simulink model "AR_Drone_Flight_Control"  (R2014a)
settings: configuration reference "AR_Drone_ConfigSet" (kept outside this file)
values from neighbouring files (symbols this model uses):
  Accelerometer_quick_calibration = [0.003485 0.008674 -0.9985]    [Calibration_Parameters.mat]
  Gyrometer_quick_calibration = [-10.63 2.778 -0.1868]    [Calibration_Parameters.mat]
undefined symbols (not defined in the file or in its folder): Accelerometer_360deg_calibration, Drone_StateModeType, Magnetometer_calibration, Navigation, Navigation_KF_Lib, sigbuilder_block
libraries: simulink x15, vrlib x7, aerolibtransform2 x5, AR_Drone_2_Library x4, dspnetwork x3, aerolibutil x2
(part 3 of 3)

== system AR_Drone_Flight_Control/Navigation/Data Conversion and Measurement Calculation/Calculate Gravity Vector/Calibration_GainOffset ==
  Pre : Inport
  Accel_Calib_Gain : Constant  Value=Accelerometer_360deg_calibration.Gains
      settings: AttributesFormatString=%<Value>
  Accel_Calib_Offset : Constant  Value=Accelerometer_360deg_calibration.Offsets
      settings: AttributesFormatString=%<Value>
  Gain : Gain  Gain=-1  OutDataTypeStr=Inherit: Same as input
  Multiply : Product  Inputs=*/
  Sum : Sum  Inputs=|+-
  Post : Outport
  wires:
  Gain/1 -> Multiply/2
  Accel_Calib_Gain/1 -> Gain/1
  Pre/1 -> Sum/1
  Sum/1 -> Multiply/1
  Accel_Calib_Offset/1 -> Sum/2
  Multiply/1 -> Post/1

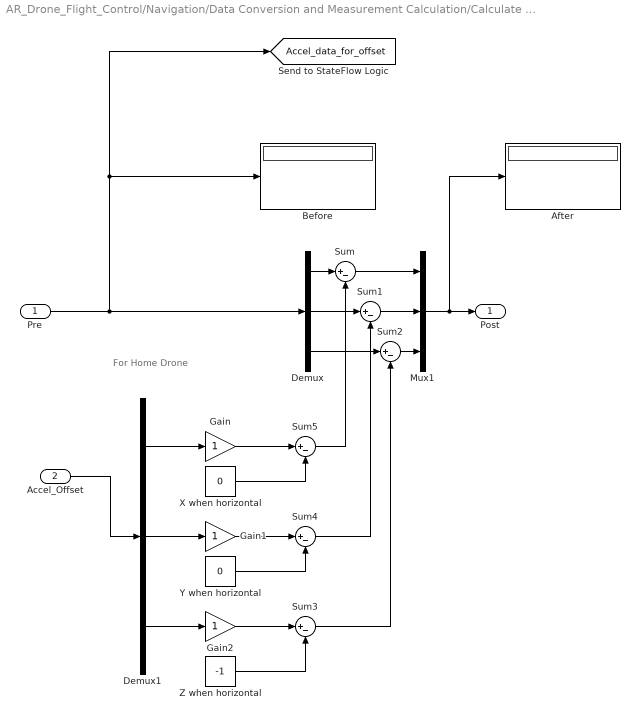
== system AR_Drone_Flight_Control/Navigation/Data Conversion and Measurement Calculation/Calculate Gravity Vector/InitialCondition_Offset ==
  note: For Home Drone
  Pre : Inport
  Accel_Offset : Inport  Port=2
  After : Display
  Before : Display
  Demux : Demux  Outputs=3
  Demux1 : Demux  Outputs=3
  Gain : Gain
  Gain1 : Gain
  Gain2 : Gain
  Mux1 : Mux  Inputs=3
  Sum{,1..5} (6 alike) : Sum  Inputs=|+-
  X when horizontal : Constant  Value=0
  Y when horizontal : Constant  Value=0
  Z when horizontal : Constant  Value=-1
  Post : Outport
  tag scope: Accel_data_for_offset=global
  wires:
  Demux1/3 -> Gain2/1
  Pre/1 -> [Accel_data_for_offset], Before/1, Demux/1
  Demux1/2 -> Gain1/1
  Demux1/1 -> Gain/1
  Accel_Offset/1 -> Demux1/1
  Mux1/1 -> After/1, Post/1
  Demux/2 -> Sum1/1
  Demux/1 -> Sum/1
  Sum1/1 -> Mux1/2
  Demux/3 -> Sum2/1
  Sum2/1 -> Mux1/3
  Sum/1 -> Mux1/1
  Gain2/1 -> Sum3/1
  Sum3/1 -> Sum2/2
  Gain1/1 -> Sum4/1
  Sum4/1 -> Sum1/2
  Gain/1 -> Sum5/1
  Sum5/1 -> Sum/2
  X when horizontal/1 -> Sum5/2
  Y when horizontal/1 -> Sum4/2
  Z when horizontal/1 -> Sum3/2

== system AR_Drone_Flight_Control/Navigation/Data Conversion and Measurement Calculation/Calculate Gravity Vector/Low Pass Filter ==
  Offset Accel : Inport
  Add : Sum
  Gain : Gain  Gain=0.8
  Gain1 : Gain  Gain=0.2
  Unit Delay : UnitDelay  SampleTime=-1
  Filtered Accel : Outport
  wires:
  Offset Accel/1 -> Gain1/1
  Add/1 -> Filtered Accel/1, Unit Delay/1
  Gain/1 -> Add/2
  Gain1/1 -> Add/1
  Unit Delay/1 -> Gain/1

== system AR_Drone_Flight_Control/Navigation/Data Conversion and Measurement Calculation/Calibration_Scale_and_Offset/Process Raw Mag Data ==
  Magnetometer : Inport
  Process Raw Mag Data (Home_330453) : Subsystem  VariantControl=TempVariantA
  Process Raw Mag Data (Work_255725) : Subsystem  VariantControl=TempVariantB
  MagVector : Outport

== system AR_Drone_Flight_Control/Navigation/Data Conversion and Measurement Calculation/Remove Offset/Process Raw Rate Gyro Data ==
  note: const float Sensitivity[ 3 ] = { 0.0609 , 0.0609 , 0.0609 } ;
      | const float Neutral[ 3 ] = { 0.0 , 0.0 , 0.0 } ;
      | const int16_t Offset[ 3 ] = { - 73 , 14 , - 13 } ;
      | const int16_t Noises[ 3 ] = { 35 , 35 , 15 } ;
      |
      | int16_t vRaws[ 3 ] = {
      | Navdata :: IMU :: Gyroscope :: getRawX (),
      | Navdata :: IMU :: Gyroscope :: getRawY (),
      | Navdata :: IMU :: Gyroscope :: getRawZ ()
      | } ;
      |
      | gyroscope[i] = vRaws[i] * Gyroscope :: Sensitivity[i] * M_PI / 180.0 ;
  Raw Rate Gyro Data : Inport
  Gain : Gain  Gain=[0.0609, 0.0609, 0.0609]  ParamDataTypeStr=double
  Processed Data : Outport
  wires:
  Gain/1 -> Processed Data/1
  Raw Rate Gyro Data/1 -> Gain/1

== system AR_Drone_Flight_Control/Navigation/SL3D Visualization/Interchange Axes Mag for SL3D /Home Drone ==
  note: z
  note: x
  note: y
  note: This comes close, however, it doesnt seem that the axis changes properly
      | ie: i rotate drone, the green dot follows it. This  tells me the Z-axis is not
      |  properly placed
  In1 : Inport
  Demux1 : Demux  Outputs=3
  Gain : Gain  Gain=-1
  Gain1 : Gain
  Gain2 : Gain
  Mux2 : Mux  Inputs=3
  Out1 : Outport
  wires:
  Gain1/1 -> Mux2/1
  Demux1/2 -> Gain1/1
  Gain/1 -> Mux2/3
  Demux1/1 -> Gain/1
  Gain2/1 -> Mux2/2
  Demux1/3 -> Gain2/1
  In1/1 -> Demux1/1
  Mux2/1 -> Out1/1

== system AR_Drone_Flight_Control/Navigation/SL3D Visualization/Interchange Axes Mag for SL3D /Subsystem ==
  note: z
  note: x
  note: y
  note: This comes close, however, it doesnt seem that the axis changes properly
      | ie: i rotate drone, the green dot follows it. This  tells me the Z-axis is not
      |  properly placed
  In1 : Inport
  Demux1 : Demux  Outputs=3
  Gain : Gain
  Gain1 : Gain  Gain=-1
  Gain2 : Gain  Gain=-1
  Mux2 : Mux  Inputs=3
  Out1 : Outport
  wires:
  In1/1 -> Demux1/1
  Demux1/3 -> Gain/1
  Demux1/2 -> Gain1/1
  Mux2/1 -> Out1/1
  Gain1/1 -> Mux2/1
  Gain/1 -> Mux2/3
  Gain2/1 -> Mux2/2
  Demux1/1 -> Gain2/1

== system AR_Drone_Flight_Control/Navigation/SL3D Visualization/Interchange Axes Mag for SL3D /Work Drone ==
  note: z
  note: x
  note: y
  note: This comes close, however, it doesnt seem that the axis changes properly
      | ie: i rotate drone, the green dot follows it. This  tells me the Z-axis is not
      |  properly placed
  In1 : Inport
  Demux1 : Demux  Outputs=3
  Gain : Gain  Gain=-1
  Gain1 : Gain
  Gain2 : Gain
  Mux2 : Mux  Inputs=3
  Out1 : Outport
  wires:
  Gain1/1 -> Mux2/1
  Demux1/2 -> Gain1/1
  Gain/1 -> Mux2/3
  Demux1/1 -> Gain/1
  Gain2/1 -> Mux2/2
  Demux1/3 -> Gain2/1
  In1/1 -> Demux1/1
  Mux2/1 -> Out1/1

== system AR_Drone_Flight_Control/Navigation/SL3D Visualization/Interchange Axes Mag for SL3D /Work Drone - supposed work drone .. not really ==
  note: z
  note: x
  note: y
  note: This comes close, however, it doesnt seem that the axis changes properly
      | ie: i rotate drone, the green dot follows it. This  tells me the Z-axis is not
      |  properly placed
  In1 : Inport
  Demux1 : Demux  Outputs=3
  Gain : Gain  Gain=-1
  Gain1 : Gain
  Gain2 : Gain  Gain=-1
  Mux2 : Mux  Inputs=3
  Out1 : Outport
  wires:
  Gain1/1 -> Mux2/1
  Demux1/2 -> Gain1/1
  Gain/1 -> Mux2/3
  Demux1/1 -> Gain/1
  Gain2/1 -> Mux2/2
  Demux1/3 -> Gain2/1
  In1/1 -> Demux1/1
  Mux2/1 -> Out1/1

== system AR_Drone_Flight_Control/Navigation/CheckSum Pre-Processing/Accelerometer Processing/CheckSum Correction/Generate Sample Holding Pulse ==
  CheckSumFlag : Inport
  HoldDataTicks_Value : Inport  Port=2
  Chart : Stateflow chart  TreatAsAtomicUnit=on
  Constant2 : Constant
  Logical Operator1 : Logic  AllPortsSameDT=off  OutDataTypeStr=boolean
  Transition Logic Detection : Subsystem
  Hold_Data_Pulse : Outport
  wires:
  HoldDataTicks_Value/1 -> Chart/2(HoldDataTicks)
  CheckSumFlag/1 -> Transition Logic Detection/1(Input)
  Transition Logic Detection/1(Transition Detect) -> Chart/1(if_transition)
  Chart/1(output) -> Logical Operator1/2
  Logical Operator1/1 -> Hold_Data_Pulse/1
  Constant2/1 -> Logical Operator1/1

== system AR_Drone_Flight_Control/Navigation/CheckSum Pre-Processing/Magnetometer/CheckSum Correction/Generate Sample Holding Pulse ==
  CheckSumFlag : Inport
  HoldDataTicks_Value : Inport  Port=2
  Chart : Stateflow chart  TreatAsAtomicUnit=on
  Constant2 : Constant
  Logical Operator1 : Logic  AllPortsSameDT=off  OutDataTypeStr=boolean
  Transition Logic Detection : Subsystem
  Hold_Data_Pulse : Outport
  wires:
  HoldDataTicks_Value/1 -> Chart/2(HoldDataTicks)
  CheckSumFlag/1 -> Transition Logic Detection/1(Input)
  Transition Logic Detection/1(Transition Detect) -> Chart/1(if_transition)
  Chart/1(output) -> Logical Operator1/2
  Logical Operator1/1 -> Hold_Data_Pulse/1
  Constant2/1 -> Logical Operator1/1

== system AR_Drone_Flight_Control/Navigation/CheckSum Pre-Processing/RateGyro Processing/CheckSum Correction/Generate Sample Holding Pulse ==
  CheckSumFlag : Inport
  HoldDataTicks_Value : Inport  Port=2
  Chart : Stateflow chart  TreatAsAtomicUnit=on
  Constant2 : Constant
  Logical Operator1 : Logic  AllPortsSameDT=off  OutDataTypeStr=boolean
  Transition Logic Detection : Subsystem
  Hold_Data_Pulse : Outport
  wires:
  HoldDataTicks_Value/1 -> Chart/2(HoldDataTicks)
  CheckSumFlag/1 -> Transition Logic Detection/1(Input)
  Transition Logic Detection/1(Transition Detect) -> Chart/1(if_transition)
  Chart/1(output) -> Logical Operator1/2
  Logical Operator1/1 -> Hold_Data_Pulse/1
  Constant2/1 -> Logical Operator1/1

== system AR_Drone_Flight_Control/Navigation/CheckSum Pre-Processing/TempFilter/CheckSum Correction/Generate Sample Holding Pulse ==
  CheckSumFlag : Inport
  HoldDataTicks_Value : Inport  Port=2
  Chart : Stateflow chart  TreatAsAtomicUnit=on
  Constant2 : Constant
  Logical Operator1 : Logic  AllPortsSameDT=off  OutDataTypeStr=boolean
  Transition Logic Detection : Subsystem
  Hold_Data_Pulse : Outport
  wires:
  HoldDataTicks_Value/1 -> Chart/2(HoldDataTicks)
  CheckSumFlag/1 -> Transition Logic Detection/1(Input)
  Transition Logic Detection/1(Transition Detect) -> Chart/1(if_transition)
  Chart/1(output) -> Logical Operator1/2
  Logical Operator1/1 -> Hold_Data_Pulse/1
  Constant2/1 -> Logical Operator1/1

== system AR_Drone_Flight_Control/Navigation/CheckSum Pre-Processing/Ultrasound Processing/CheckSum Correction/Generate Sample Holding Pulse ==
  CheckSumFlag : Inport
  HoldDataTicks_Value : Inport  Port=2
  Chart : Stateflow chart  TreatAsAtomicUnit=on
  Constant2 : Constant
  Logical Operator1 : Logic  AllPortsSameDT=off  OutDataTypeStr=boolean
  Transition Logic Detection : Subsystem
  Hold_Data_Pulse : Outport
  wires:
  HoldDataTicks_Value/1 -> Chart/2(HoldDataTicks)
  CheckSumFlag/1 -> Transition Logic Detection/1(Input)
  Transition Logic Detection/1(Transition Detect) -> Chart/1(if_transition)
  Chart/1(output) -> Logical Operator1/2
  Logical Operator1/1 -> Hold_Data_Pulse/1
  Constant2/1 -> Logical Operator1/1

== system AR_Drone_Flight_Control/Navigation/Data Conversion and Measurement Calculation/Calibration_Scale_and_Offset/Process Raw Mag Data/Process Raw Mag Data (Home_330453) ==
  note: magnetometer[ 0 ] = - ( float ) navdata.mx ;
      | magnetometer[ 1 ] = ( float ) navdata.my ;
      | magnetometer[ 2 ] = - ( float ) navdata.mz ;
      | const float Sensitivity[ 3 ] = { 0.0071492608 , 0.0070882491 , 0.0074057781 } ;
      | const float Neutral[ 3 ] = { 118.0 , - 65.0 , 110.0 } ;
  Magnetometer : Inport
  Bias : Constant  Commented=on  Value=[-23 4.3 1.44]
  Constant : Constant  Value=Magnetometer_calibration.Offsets
      settings: AttributesFormatString=%<Value>
  Constant1 : Constant  Value=Magnetometer_calibration.Gains
      settings: AttributesFormatString=%<Value>
  Divide : Product  Inputs=/*
  Sum : Sum  Inputs=|+-
  postGain : Gain  Commented=on  Gain=1./[187 163 139]
  MagVector : Outport
  wires:
  Constant1/1 -> Divide/1
  Sum/1 -> Divide/2
  Magnetometer/1 -> Sum/1
  Constant/1 -> Sum/2
  Divide/1 -> MagVector/1

== system AR_Drone_Flight_Control/Navigation/Data Conversion and Measurement Calculation/Calibration_Scale_and_Offset/Process Raw Mag Data/Process Raw Mag Data (Work_255725) ==
  note: 158 145 136
  note: magnetometer[ 0 ] = - ( float ) navdata.mx ;
      | magnetometer[ 1 ] = ( float ) navdata.my ;
      | magnetometer[ 2 ] = - ( float ) navdata.mz ;
      | const float Sensitivity[ 3 ] = { 0.0071492608 , 0.0070882491 , 0.0074057781 } ;
      | const float Neutral[ 3 ] = { 118.0 , - 65.0 , 110.0 } ;
  Magnetometer : Inport
  Bias : Constant  Value=[2.93 18.9 77.5]
  Low Pass Filter1 : Subsystem  Commented=through
      mask Display: disp(['Elliptic Filter with 20 Hz corner', '\n', '44 dB stopband.'])
  Sum : Sum  Inputs=|+-
  postGain : Gain  Gain=1./[167 135 132]
  preGain : Gain  Commented=through  Gain=[1 1 1]
  MagVector : Outport
  wires:
  postGain/1 -> Low Pass Filter1/1(Input)
  Magnetometer/1 -> preGain/1
  Sum/1 -> postGain/1
  preGain/1 -> Sum/1
  Bias/1 -> Sum/2
  Low Pass Filter1/1(Output) -> MagVector/1

== system AR_Drone_Flight_Control/Navigation/CheckSum Pre-Processing/Accelerometer Processing/CheckSum Correction/Generate Sample Holding Pulse/Transition Logic Detection ==
  Input : Inport
  Constant : Constant  Value=0
  Constant1 : Constant
  Logical Operator : Logic  AllPortsSameDT=off  OutDataTypeStr=boolean
  Relational Operator : RelationalOperator  Operator===  OutDataTypeStr=boolean
  Relational Operator1 : RelationalOperator  Operator===  OutDataTypeStr=boolean
  Unit Delay : UnitDelay  SampleTime=-1
  Transition Detect : Outport
  wires:
  Logical Operator/1 -> Transition Detect/1  "Transition_Detect"
  Constant1/1 -> Relational Operator1/1
  Constant/1 -> Relational Operator/2
  Relational Operator/1 -> Logical Operator/2
  Input/1 -> Unit Delay/1, Relational Operator1/2
  Unit Delay/1 -> Relational Operator/1
  Relational Operator1/1 -> Logical Operator/1

== system AR_Drone_Flight_Control/Navigation/CheckSum Pre-Processing/Magnetometer/CheckSum Correction/Generate Sample Holding Pulse/Transition Logic Detection ==
  Input : Inport
  Constant : Constant  Value=0
  Constant1 : Constant
  Logical Operator : Logic  AllPortsSameDT=off  OutDataTypeStr=boolean
  Relational Operator : RelationalOperator  Operator===  OutDataTypeStr=boolean
  Relational Operator1 : RelationalOperator  Operator===  OutDataTypeStr=boolean
  Unit Delay : UnitDelay  SampleTime=-1
  Transition Detect : Outport
  wires:
  Logical Operator/1 -> Transition Detect/1  "Transition_Detect"
  Constant1/1 -> Relational Operator1/1
  Constant/1 -> Relational Operator/2
  Relational Operator/1 -> Logical Operator/2
  Input/1 -> Unit Delay/1, Relational Operator1/2
  Unit Delay/1 -> Relational Operator/1
  Relational Operator1/1 -> Logical Operator/1

== system AR_Drone_Flight_Control/Navigation/CheckSum Pre-Processing/RateGyro Processing/CheckSum Correction/Generate Sample Holding Pulse/Transition Logic Detection ==
  Input : Inport
  Constant : Constant  Value=0
  Constant1 : Constant
  Logical Operator : Logic  AllPortsSameDT=off  OutDataTypeStr=boolean
  Relational Operator : RelationalOperator  Operator===  OutDataTypeStr=boolean
  Relational Operator1 : RelationalOperator  Operator===  OutDataTypeStr=boolean
  Unit Delay : UnitDelay  SampleTime=-1
  Transition Detect : Outport
  wires:
  Logical Operator/1 -> Transition Detect/1  "Transition_Detect"
  Constant1/1 -> Relational Operator1/1
  Constant/1 -> Relational Operator/2
  Relational Operator/1 -> Logical Operator/2
  Input/1 -> Unit Delay/1, Relational Operator1/2
  Unit Delay/1 -> Relational Operator/1
  Relational Operator1/1 -> Logical Operator/1

== system AR_Drone_Flight_Control/Navigation/CheckSum Pre-Processing/TempFilter/CheckSum Correction/Generate Sample Holding Pulse/Transition Logic Detection ==
  Input : Inport
  Constant : Constant  Value=0
  Constant1 : Constant
  Logical Operator : Logic  AllPortsSameDT=off  OutDataTypeStr=boolean
  Relational Operator : RelationalOperator  Operator===  OutDataTypeStr=boolean
  Relational Operator1 : RelationalOperator  Operator===  OutDataTypeStr=boolean
  Unit Delay : UnitDelay  SampleTime=-1
  Transition Detect : Outport
  wires:
  Logical Operator/1 -> Transition Detect/1  "Transition_Detect"
  Constant1/1 -> Relational Operator1/1
  Constant/1 -> Relational Operator/2
  Relational Operator/1 -> Logical Operator/2
  Input/1 -> Unit Delay/1, Relational Operator1/2
  Unit Delay/1 -> Relational Operator/1
  Relational Operator1/1 -> Logical Operator/1

== system AR_Drone_Flight_Control/Navigation/CheckSum Pre-Processing/Ultrasound Processing/CheckSum Correction/Generate Sample Holding Pulse/Transition Logic Detection ==
  Input : Inport
  Constant : Constant  Value=0
  Constant1 : Constant
  Logical Operator : Logic  AllPortsSameDT=off  OutDataTypeStr=boolean
  Relational Operator : RelationalOperator  Operator===  OutDataTypeStr=boolean
  Relational Operator1 : RelationalOperator  Operator===  OutDataTypeStr=boolean
  Unit Delay : UnitDelay  SampleTime=-1
  Transition Detect : Outport
  wires:
  Logical Operator/1 -> Transition Detect/1  "Transition_Detect"
  Constant1/1 -> Relational Operator1/1
  Constant/1 -> Relational Operator/2
  Relational Operator/1 -> Logical Operator/2
  Input/1 -> Unit Delay/1, Relational Operator1/2
  Unit Delay/1 -> Relational Operator/1
  Relational Operator1/1 -> Logical Operator/1

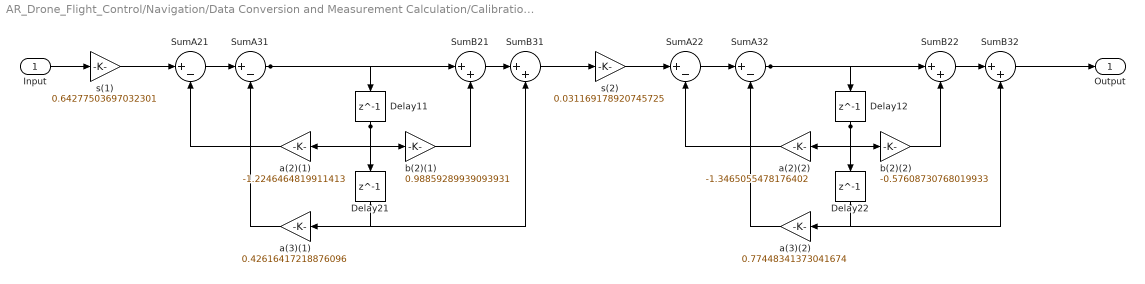
== system AR_Drone_Flight_Control/Navigation/Data Conversion and Measurement Calculation/Calibration_Scale_and_Offset/Process Raw Mag Data/Process Raw Mag Data (Work_255725)/Low Pass Filter1 ==
  Input : Inport
  Delay{11..12,21..22} (4 alike) : Delay  DelayLength=1  InitialCondition=0
  SumA{21..22,31..32} (4 alike) : Sum  Inputs=|+-  RndMeth=Nearest  SaturateOnIntegerOverflow=on  OutDataTypeStr=Inherit: Same as first input
  SumB{21..22,31..32} (4 alike) : Sum  Inputs=|++  RndMeth=Nearest  SaturateOnIntegerOverflow=on  OutDataTypeStr=Inherit: Same as first input
  a(2)(1) : Gain  Gain=-1.2246464819911413  ParamDataTypeStr=double  RndMeth=Nearest  SaturateOnIntegerOverflow=on  OutDataTypeStr=Inherit: Same as input
  a(2)(2) : Gain  Gain=-1.3465055478176402  ParamDataTypeStr=double  RndMeth=Nearest  SaturateOnIntegerOverflow=on  OutDataTypeStr=Inherit: Same as input
  a(3)(1) : Gain  Gain=0.42616417218876096  ParamDataTypeStr=double  RndMeth=Nearest  SaturateOnIntegerOverflow=on  OutDataTypeStr=Inherit: Same as input
  a(3)(2) : Gain  Gain=0.77448341373041674  ParamDataTypeStr=double  RndMeth=Nearest  SaturateOnIntegerOverflow=on  OutDataTypeStr=Inherit: Same as input
  b(2)(1) : Gain  Gain=0.98859289939093931  ParamDataTypeStr=double  RndMeth=Nearest  SaturateOnIntegerOverflow=on  OutDataTypeStr=Inherit: Same as input
  b(2)(2) : Gain  Gain=-0.57608730768019933  ParamDataTypeStr=double  RndMeth=Nearest  SaturateOnIntegerOverflow=on  OutDataTypeStr=Inherit: Same as input
  s(1) : Gain  Gain=0.64277503697032301  ParamDataTypeStr=double  RndMeth=Nearest  SaturateOnIntegerOverflow=on  OutDataTypeStr=Inherit: Same as input
  s(2) : Gain  Gain=0.031169178920745725  ParamDataTypeStr=double  RndMeth=Nearest  SaturateOnIntegerOverflow=on  OutDataTypeStr=Inherit: Same as input
  Output : Outport
  wires:
  Delay22/1 -> SumB32/2, a(3)(2)/1
  a(3)(2)/1 -> SumA32/2
  b(2)(2)/1 -> SumB22/2
  Delay12/1 -> Delay22/1, b(2)(2)/1, a(2)(2)/1
  a(2)(2)/1 -> SumA22/2
  SumB32/1 -> Output/1
  SumB22/1 -> SumB32/1
  SumA32/1 -> Delay12/1, SumB22/1
  SumA22/1 -> SumA32/1
  s(2)/1 -> SumA22/1
  Delay21/1 -> SumB31/2, a(3)(1)/1
  a(3)(1)/1 -> SumA31/2
  b(2)(1)/1 -> SumB21/2
  Delay11/1 -> Delay21/1, b(2)(1)/1, a(2)(1)/1
  a(2)(1)/1 -> SumA21/2
  SumB31/1 -> s(2)/1
  SumB21/1 -> SumB31/1
  SumA31/1 -> Delay11/1, SumB21/1
  SumA21/1 -> SumA31/1
  s(1)/1 -> SumA21/1
  Input/1 -> s(1)/1

== stateflow chart AR_Drone_Flight_Control/Navigation/CheckSum Pre-Processing/Accelerometer Processing/CheckSum Correction/Generate Sample Holding Pulse/Chart ==
  state Begin_State0
    entry: output =0;
  state Begin_State
    entry: output =1;
  state End_State
    entry: output=0;
  (default) -> Begin_State0
  Begin_State0 -> Begin_State : [if_transition==1]
  Begin_State -> End_State [order 1] : after(HoldDataTicks,tick)
  End_State -> Begin_State : [if_transition==1]
  Begin_State -> Begin_State [order 2] : [if_transition==1]
  data: output output; if_transition input; HoldDataTicks input

== stateflow chart AR_Drone_Flight_Control/Navigation/CheckSum Pre-Processing/RateGyro Processing/CheckSum Correction/Generate Sample Holding Pulse/Chart ==
  state Begin_State0
    entry: output =0;
  state Begin_State
    entry: output =1;
  state End_State
    entry: output=0;
  (default) -> Begin_State0
  Begin_State0 -> Begin_State : [if_transition==1]
  Begin_State -> End_State [order 1] : after(HoldDataTicks,tick)
  End_State -> Begin_State : [if_transition==1]
  Begin_State -> Begin_State [order 2] : [if_transition==1]
  data: output output; if_transition input; HoldDataTicks input

== stateflow chart AR_Drone_Flight_Control/Navigation/CheckSum Pre-Processing/Magnetometer/CheckSum Correction/Generate Sample Holding Pulse/Chart ==
  state Begin_State0
    entry: output =0;
  state Begin_State
    entry: output =1;
  state End_State
    entry: output=0;
  (default) -> Begin_State0
  Begin_State0 -> Begin_State : [if_transition==1]
  Begin_State -> End_State [order 1] : after(HoldDataTicks,tick)
  End_State -> Begin_State : [if_transition==1]
  Begin_State -> Begin_State [order 2] : [if_transition==1]
  data: output output; if_transition input; HoldDataTicks input

== stateflow chart AR_Drone_Flight_Control/Navigation/CheckSum Pre-Processing/TempFilter/CheckSum Correction/Generate Sample Holding Pulse/Chart ==
  state Begin_State0
    entry: output =0;
  state Begin_State
    entry: output =1;
  state End_State
    entry: output=0;
  (default) -> Begin_State0
  Begin_State0 -> Begin_State : [if_transition==1]
  Begin_State -> End_State [order 1] : after(HoldDataTicks,tick)
  End_State -> Begin_State : [if_transition==1]
  Begin_State -> Begin_State [order 2] : [if_transition==1]
  data: output output; if_transition input; HoldDataTicks input

== matlab function AR_Drone_Flight_Control/Data decomposition to 3D Visualization/SL3D Visualization1/Matrix Re-Order ==
  data: M_in input; M_out output
function M_out = MatrixFormat(M_in)
%#codegen

% SL3D coordinate system is different. This EML block is responsible for
% re-ordering the matrix in a format that SL3D can understand

M_out = M_in ; %set size

%re-order diagonal
M_out(1,1) = M_in(2,2);
M_out(2,2) = M_in(3,3);
M_out(3,3) = M_in(1,1);

%re-order bottom half
M_out(2,1) = M_in(3,2) ;
M_out(3,1) = M_in(1,2) ;
M_out(3,2) = M_in(1,3);

%re-order upper half
M_out(1,2) = M_in(2,3);
M_out(1,3) = M_in(2,1) ;
M_out(2,3) = M_in(3,1);

== matlab function AR_Drone_Flight_Control/Flight Controller/Supervisory Flight Controller/Attitude_Control/MATLAB Function ==
  data: error input; err_normalized output
function err_normalized = normalize_angle(error)
%#codegen

err_normalized = error;

% limit the yaw component to +/- 180 degrees
% if (error(3) > 180)    % Normalize to -180,180
%     err_normalized(3) = error(3) - 360;
% elseif(error(3) < -180)
%     err_normalized(3) = error(3) + 360;
% end

end

== matlab function AR_Drone_Flight_Control/Navigation/SL3D Visualization/Matrix Re-Order ==
  data: M_in input; M_out output
function M_out = MatrixFormat(M_in)
%#codegen

% SL3D coordinate system is different. This EML block is responsible for
% re-ordering the matrix in a format that SL3D can understand

M_out = M_in ; %set size

%re-order diagonal
M_out(1,1) = M_in(2,2);
M_out(2,2) = M_in(3,3);
M_out(3,3) = M_in(1,1);

%re-order bottom half
M_out(2,1) = M_in(3,2) ;
M_out(3,1) = M_in(1,2) ;
M_out(3,2) = M_in(1,3);

%re-order upper half
M_out(1,2) = M_in(2,3);
M_out(1,3) = M_in(2,1) ;
M_out(2,3) = M_in(3,1);

== matlab function AR_Drone_Flight_Control/Flight Controller/Supervisory Flight Controller/Motor_Mixing/RampDownInSpeed1 ==
  data: Cmd input; motorCmd output; stopCmd input
function motorCmd = fcn(Cmd,stopCmd)
%#codegen
persistent tempCmd;
if(isempty(tempCmd))
    tempCmd = ([0;0;0;0]);
end
if(stopCmd)
    tempCmd = tempCmd + ([1;1;1;1]*15/400);
    motorCmd = Cmd - tempCmd;
    
else
    tempCmd = ([0;0;0;0]);
    motorCmd = Cmd;
end

% if (motorCmd(1) <=0)
%         motorCmd = ([0;0;0;0]);
% end

%apply lower bounding
for i=1:4
    
if motorCmd(i)<0
    motorCmd(i) = 0;
end

end
